simulink model "Digital_PID_controller"  (R2023b)
settings: Solver=VariableStepAuto  StartTime=0.0  StopTime=10.0  RelTol=1e-3
settings Model: Creator=gaafa  LastModifiedBy=gaafa

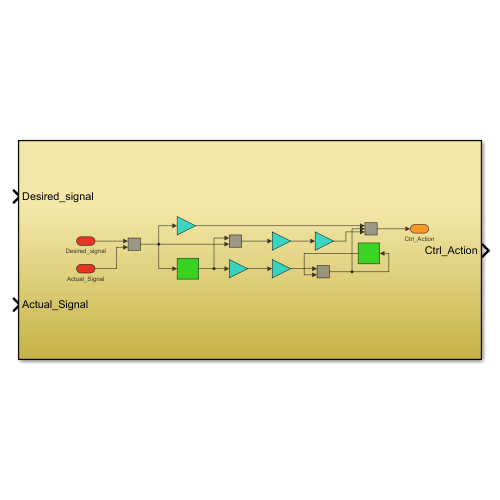
[thumbnail: Simulink's stored preview of the top-level diagram]
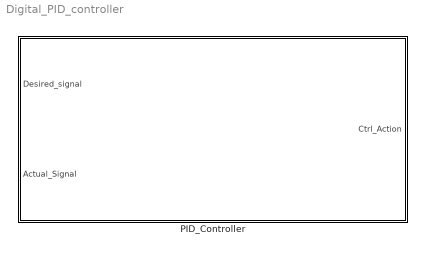
== system Digital_PID_controller ==
  PID_Controller : Subsystem

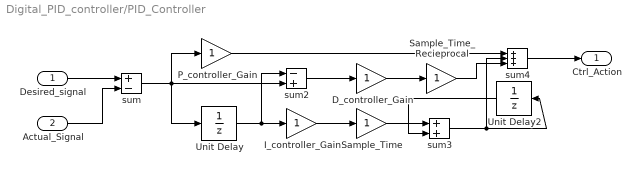
== system Digital_PID_controller/PID_Controller ==
  Desired_signal : Inport
  Actual_Signal : Inport  Port=2
  D_controller_Gain : Gain
  I_controller_Gain : Gain
  P_controller_Gain : Gain
  Sample_Time : Gain
  Sample_Time_Recieprocal : Gain
  Unit Delay : UnitDelay  SampleTime=-1  HasFrameUpgradeWarning=on
  Unit Delay2 : UnitDelay  SampleTime=-1  HasFrameUpgradeWarning=on
  sum : Sum  Inputs=+-
  sum2 : Sum  Inputs=-+
  sum3 : Sum
  sum4 : Sum  Inputs=+++
  Ctrl_Action : Outport
  wires:
  Unit Delay2/1 -> sum3/2
  Desired_signal/1 -> sum/1
  sum4/1 -> Ctrl_Action/1
  Actual_Signal/1 -> sum/2
  sum/1 -> sum2/2, P_controller_Gain/1, Unit Delay/1
  P_controller_Gain/1 -> sum4/1
  Unit Delay/1 -> I_controller_Gain/1, sum2/1
  sum2/1 -> D_controller_Gain/1
  D_controller_Gain/1 -> Sample_Time_Recieprocal/1
  I_controller_Gain/1 -> Sample_Time/1
  Sample_Time_Recieprocal/1 -> sum4/3
  Sample_Time/1 -> sum3/1
  sum3/1 -> Unit Delay2/1, sum4/2
